simulink model "Non_Holonomical_Cubli"  (R2025b)
settings: Solver=ode15s  StartTime=0  StopTime=13  MaxStep=1e-3  MinStep=1e-8  RelTol=1e-3
values from neighbouring files (symbols this model uses):
  m = 1.219    [physical_parameters.mat]    (also in tuning_parameter_corner.mat; tuning_parameter_edge.mat)
undefined symbols (not defined in the file or in its folder): X, Y, Z
libraries: sm_lib x79, nesl_utility x10, simulink x5, simulink_extras x2
(part 3 of 3)

== system Non_Holonomical_Cubli/Cubli System/Cubli/Non-Motor frame setup/Nonmotor frame 3/Frame ==
  Regular frame : sm_lib/Body Elements/File Solid  ExtGeomFileName=D:\Mechatronics\Non-Holonomical Cubli\GitHub Referance\balancing-cube-main\mechanical\models\frame-regular.step  UnitType=FromFile  ExtGeomFileUnits=m  StepReaderType=HEX  ExportConvexHullGeometry=off  InertiaType=Custom  BasedOnType=DensityFromFile  Density=1000  DensityUnits=kg/m^3  Mass=27.912  MassUnits=g  CenterOfMass=[75.00 75.00 1.481]  CenterOfMassUnits=mm  MomentsOfInertia=[8.5196926e-5 5.2659387e-5 1.378e-4]  MomentsOfInertiaUnits=kg*m^2  ProductsOfInertia=[0 0 0]  ProductsOfInertiaUnits=kg*m^2  GraphicType=FromGeometry  MarkerShape=Sphere  MarkerSize=10  GraphicVisPropType=SimpleVisualProperties  GraphicDiffuseColor=[0 0.5137 0.8314]  GraphicOpacity=1  GraphicSpecularColor=[0.5 0.5 0.5 1.0]  GraphicAmbientColor=[0.15 0.15 0.15 1.0]  GraphicEmissiveColor=[0.0 0.0 0.0 1.0]  GraphicShininess=75  DoExposeReferenceFrame=on  SerializedFrames=<Frames/>
  World to frame : sm_lib/Frames and Transforms/Rigid Transform  RotationMethod=None  FollAlignAxisA=+X  BaseAlignAxisA=+Y  FollAlignAxisB=+Y  BaseAlignAxisB=+Z  RotationStandardAxis=+Z  RotationAngle=0  RotationAngleUnits=deg  RotationArbitraryAxis=[0 0 1]  RotationSequenceAxes=FollowerAxes  RotationSequence=XYX  RotationSequenceAngles=[0 0 0]  RotationSequenceAnglesUnits=deg  RotationMatrix=[1 0 0;0 1 0;0 0 1]  Quaternion=[1 0 0 0]  TranslationMethod=Cartesian  TranslationCartesianOffset=[-75 -75 0]  TranslationCartesianOffsetUnits=mm  TranslationStandardAxis=+Z  TranslationStandardOffset=7  TranslationStandardOffsetUnits=mm  TranslationROffset=0  TranslationROffsetUnits=m  TranslationThetaOffset=0  TranslationThetaOffsetUnits=deg  TranslationZOffset=0  TranslationZOffsetUnits=m
  W to F : PMIOPort  Side=Left
  connections:
  W to F/RConn1 -- World to frame/LConn1
  Regular frame/RConn1 -- World to frame/RConn1

== system Non_Holonomical_Cubli/Cubli System/Cubli/Non-Motor frame setup/Nonmotor frame 3/PCB setup ==
  Frame to PCB : sm_lib/Frames and Transforms/Rigid Transform  RotationMethod=None  FollAlignAxisA=+X  BaseAlignAxisA=+Y  FollAlignAxisB=+Y  BaseAlignAxisB=+Z  RotationStandardAxis=+Z  RotationAngle=0  RotationAngleUnits=deg  RotationArbitraryAxis=[0 0 1]  RotationSequenceAxes=FollowerAxes  RotationSequence=XYX  RotationSequenceAngles=[0 0 0]  RotationSequenceAnglesUnits=deg  RotationMatrix=[1 0 0;0 1 0;0 0 1]  Quaternion=[1 0 0 0]  TranslationMethod=Cartesian  TranslationCartesianOffset=[0 0 -12]  TranslationCartesianOffsetUnits=mm  TranslationStandardAxis=+Z  TranslationStandardOffset=0  TranslationStandardOffsetUnits=m  TranslationROffset=0  TranslationROffsetUnits=m  TranslationThetaOffset=0  TranslationThetaOffsetUnits=deg  TranslationZOffset=0  TranslationZOffsetUnits=m
  PCB : sm_lib/Body Elements/Brick Solid  BrickDimensions=[95 95 15]  BrickDimensionsUnits=mm  ExportEntireGeometry=off  InertiaType=CalculateFromGeometry  BasedOnType=Mass  Density=1000  DensityUnits=kg/m^3  Mass=138.5  MassUnits=g  CenterOfMass=[0 0 0]  CenterOfMassUnits=mm  MomentsOfInertia=[8.25e-5 8.25e-5 1.485e-4]  MomentsOfInertiaUnits=kg*m^2  ProductsOfInertia=[0 0 0]  ProductsOfInertiaUnits=kg*m^2  GraphicType=FromGeometry  MarkerShape=Sphere  MarkerSize=10  GraphicVisPropType=SimpleVisualProperties  GraphicDiffuseColor=[0.5922 0 0.9608]  GraphicOpacity=1  GraphicSpecularColor=[0.5 0.5 0.5 1.0]  GraphicAmbientColor=[0.15 0.15 0.15 1.0]  GraphicEmissiveColor=[0.0 0.0 0.0 1.0]  GraphicShininess=75  DoExposeReferenceFrame=on  SerializedFrames=<Frames/>
  F to P : PMIOPort  Side=Left
  connections:
  PCB/RConn1 -- Frame to PCB/RConn1
  Frame to PCB/LConn1 -- F to P/RConn1

== matlab function Non_Holonomical_Cubli/Master Controller/Corner_Balance_Torque/quaternion_corner_controller ==
  settings: sampleTime=0.00001
  data: q_current input; tau_x output; omega_frame input; omega_wheels input; jump_tigger input; tau_y output; tau_z output; tau_y_edge input; q_ev_corner output; error_distance output
function [tau_x, tau_y, tau_z, q_ev_corner, error_distance] = quaternion_corner_controller(q_current, omega_frame, omega_wheels, jump_tigger, tau_y_edge)
    % q_current:    [w, x, y, z] live orientation from the IMU/Sensor
    % omega_frame:  [wx, wy, wz] in rad/s from the gyroscope (Body Frame)
    % omega_wheels: [wx_wheel, wy_wheel, wz_wheel] in rad/s

    tau_x = 0;
    tau_y = 0;
    tau_z = 0;

    % =========================================================
    % 1. PHYSICAL CONSTANTS
    % =========================================================
    I_matrix = [0.01757, -0.00664, -0.00656; 
               -0.00664,  0.01757, -0.00656; 
               -0.00656, -0.00656,  0.01757];
               
    I_wheel = 0.0005148;     
    m = 1.219;           
    g = 9.80665;            
    r_com = [0.0724; 0.0724; 0.0724]; 

    % =========================================================
    % 2. TARGET ORIENTATIONS (Pre-calculated Quaternions)
    % =========================================================
    % A. The True Corner (Roll = 45 deg, Pitch = -35.26 deg, Yaw = 0)
    % Taken exactly from your previously successful sensor readings
    q_target_corner = [0.8805, 0.2798, -0.3647, -0.1159];
    
    % =========================================================
    % 3. ERROR CALCULATION & UNWINDING FIX (Hamilton Product)
    % =========================================================
    % Extract current quaternion components for readability
    wc = q_current(1); xc = q_current(2); yc = q_current(3); zc = q_current(4);
    
    % --- Calculate Error for the CORNER ---
    % q_error = q_target_corner_inverse * q_current
    w1_c = q_target_corner(1); x1_c = -q_target_corner(2); y1_c = -q_target_corner(3); z1_c = -q_target_corner(4);
    
    q_ew_c = w1_c*wc - x1_c*xc - y1_c*yc - z1_c*zc;
    q_ex_c = w1_c*xc + x1_c*wc + y1_c*zc - z1_c*yc;
    q_ey_c = w1_c*yc - x1_c*zc + y1_c*wc + z1_c*xc;
    q_ez_c = w1_c*zc + x1_c*yc - y1_c*xc + z1_c*wc;
    
    % Shortest path enforcement (Unwinding Fix)
    if q_ew_c < 0
        q_ew_c = -q_ew_c; q_ex_c = -q_ex_c; q_ey_c = -q_ey_c; q_ez_c = -q_ez_c;
    end
    q_ev_corner = [q_ex_c; q_ey_c; q_ez_c];
    
    % Check how close the cube is to the 3D corner (Vector Magnitude)
    error_distance = norm(q_ev_corner);

    % =========================================================
    % 4. STATE MACHINE (Edge to Corner Logic)
    % =========================================================

    if jump_tigger > 0.0 && jump_tigger < 2.0
        % ---------------------------------------------------------
        % STATE 1: THE X-AXIS TORQUE BUILD UP
        % ---------------------------------------------------------
        jump_torque_x =  0.15; % Fire the X-wheel upward
        jump_torque_z = -0.15; % Fire the Z-wheel upward
        
        tau_motor = [jump_torque_x; tau_y_edge; jump_torque_z];

        tau_x = tau_motor(1);
        tau_y = tau_motor(2);
        tau_z = tau_motor(3);

    elseif jump_tigger >= 2.0 && jump_tigger < 2.02
        % ---------------------------------------------------------
        % STATE 2: THE X-AXIS JUMP
        % ---------------------------------------------------------
        jump_torque_x = -14.5; % Fire the X-wheel upward
        jump_torque_z =  14.5; % Fire the Z-wheel upward
        
        tau_motor = [jump_torque_x; 0; jump_torque_z];

        tau_x = tau_motor(1);
        tau_y = tau_motor(2);
        tau_z = tau_motor(3);
        
    elseif jump_tigger >= 2.032 && error_distance <= 0.075

        % ---------------------------------------------------------
        % STATE 3: SMC 3D CORNER CATCH & BALANCE
        % ---------------------------------------------------------
        c = diag([30, 30, 30]);      
        K = [1.5; 1.5; 1.5];             
        epsilon = 0.1; 
        
        % A. Exact Quaternion Derivative for alpha_desired
        q_ev_dot = 0.5 * (q_ew_c * omega_frame + cross(q_ev_corner, omega_frame));
        
        % B. The 3D Sliding Surface
        S = (c * q_ev_corner) + omega_frame;
        
        % C. Dynamic Gravity Compensation (Using Quaternion to DCM rotation)
        % Extracts the 3rd Row of the rotation matrix using live quaternion values
        R31 = 2 * (xc*zc - wc*yc);
        R32 = 2 * (yc*zc + wc*xc);
        R33 = 1 - 2 * (xc^2 + yc^2);
        
        g_body_rotated = [-g * R31; -g * R32; -g * R33];
        tau_gravity = cross(r_com, m * g_body_rotated);
        
        % D. SMC Equivalent Control (tau_eq)
        L_wheels = I_wheel .* omega_wheels; 
        alpha_desired = -c * q_ev_dot;
        
        tau_eq = - (I_matrix * alpha_desired) - cross(omega_frame, (I_matrix * omega_frame + L_wheels)) - tau_gravity;
                 
        % E. SMC Switching Control (tau_sw)
        tau_sw = -K .* tanh(S / epsilon);
        
        % F. Total Torque (Newton's Third Law flipped)
        tau_frame = tau_eq + tau_sw;
        tau_motor = -tau_frame;

        % G. Motor Saturation
        max_torque = 1.2;
        tau_x = max(min(tau_motor(1), max_torque), -max_torque);
        tau_y = max(min(tau_motor(2), max_torque), -max_torque);
        tau_z = max(min(tau_motor(3), max_torque), -max_torque);
    end 
end

== matlab function Non_Holonomical_Cubli/Master Controller/Edge_Balance_Torque/Edge_SMC ==
  data: tau_x output; theta_current input; omega_frame input; omega_wheels input; tau_y output; tau_z output; error_distance output; jump_trigger input
function [tau_x, tau_y, tau_z,error_distance] = smc_edge_controller(theta_current, omega_frame, omega_wheels, jump_trigger)
    % theta_current: [roll, pitch, yaw] in radians from the sensor (Earth Frame)
    % omega_frame:   [wx, wy, wz] in rad/s from the gyroscope (Body Frame)
    % omega_wheels:  [wx_wheel, wy_wheel, wz_wheel] in rad/s

    jump_check = 0;
    tau_motor = [0; 0; 0;];

    % =========================================================
    % 1. PHYSICAL CONSTANTS (Matches your CAD parameters)
    % =========================================================
    I_matrix = [0.01757, -0.00664, -0.00656; 
               -0.00664,  0.01757, -0.00656; 
               -0.00656, -0.00656,  0.01757];
               
    I_wheel = 0.0005148;     % Inertia of a single brass wheel (kg*m^2)
    m = 1.291;           % Total mass (kg)
    g = 9.80665;            % Gravity (m/s^2)
    
    % True Center of Mass vector from the EDGE pivot
    r_com = [0.0724; 0.0724; 0.0724]; 

    % =========================================================
    % 2. OUTER LOOP: MOMENTUM MANAGEMENT (Deadband Lean)
    % =========================================================
    % We apply a proportional shift ONLY if the wheel exceeds the safe zone.
    safe_speed = 200;  % ~1000 RPM in rad/s
    k_momentum = 1e-4; % Gain: How much to lean per rad/s over the limit
    max_lean = 0.0167*3;     % Safety limit: Max lean of ~1 degrees

    % Read instantaneous Y-axis (Pitch) wheel speed
    pitch_wheel_speed = omega_wheels(2);

    % Deadband logic
    if pitch_wheel_speed > safe_speed
        active_omega = pitch_wheel_speed - safe_speed;
    elseif pitch_wheel_speed < -safe_speed
        active_omega = pitch_wheel_speed + safe_speed;
    else
        active_omega = 0; % Inside safe zone, do not lean
    end 

    % Calculate and saturate the lean shift
    lean_shift = k_momentum * active_omega;
    lean_shift = max(min(lean_shift, max_lean), -max_lean);

    % Generate dynamic target (Base -45 deg edge + shift)
    target_pitch = -0.7854 - lean_shift;
    theta_target = [0; target_pitch; 0];
    
    % =========================================================
    % 3. CALCULATE ERRORS & FRAME MAPPING
    % =========================================================
    % Raw Position error (In Earth Frame)
    e_euler = theta_current - theta_target;
    
    % Extract current Roll (phi) and Pitch (theta)
    phi = theta_current(1);
    theta = theta_current(2);
    
    % Kinematic Transformation Matrix (W)
    % Maps Earth-frame Euler angle errors into physical Body-frame axes
    W = [1,  0,        -sin(theta); 
         0,  cos(phi),  sin(phi)*cos(theta); 
         0, -sin(phi),  cos(phi)*cos(theta)];
         
    % Project the error into the physical Body Frame
    e_body = W * e_euler;
    e_dot_body = omega_frame;
    
    % Check how close the cube is to the edge balance point (in radians)
    error_distance = norm(e_body);

    % =========================================================
    % 4. SMC 3D EDGE CATCH & BALANCE
    % =========================================================
    if jump_trigger >= 0.2 && jump_trigger <= 2.3
        % ---------------------------------------------------------
        % STATE 1: THE Y-AXIS TORQUE BUILD UP
        % ---------------------------------------------------------
        tau_motor = [0; -0.2; 0];

        jump_check = 0;

    elseif jump_trigger >= 2.3 && jump_trigger <= 2.32
        % ---------------------------------------------------------
        % STATE 2: THE Y-AXIS JUMP
        % ---------------------------------------------------------
        tau_motor = [0; 21; 0];

        jump_check = 1;

    elseif jump_trigger >= 2.32 && theta <= -0.3927
        % A. SMC Tuning Parameters
        c = 30;        % Sliding surface slope (Urgency)
        K = 0.8;       % Switching gain (Muscle)
        epsilon = 0.1; % Boundary layer (Smooths out chattering)
        
        % B. The 3D Sliding Surface (3x1 Vector)
        S = (c * e_body) + e_dot_body;
        
        % C. Dynamic Gravity Compensation (Rotate World Z down to Body)
        R31 = -sin(theta);
        R32 = cos(theta) * sin(phi);
        R33 = cos(theta) * cos(phi);
        g_body_rotated = [-g * R31; -g * R32; -g * R33];
        tau_gravity = cross(r_com, m * g_body_rotated);
        
        % D. SMC Equivalent Control (tau_eq)
        L_wheels = I_wheel .* omega_wheels; 
        alpha_desired = -c * e_dot_body;
        
        % Full 3D Inverse Dynamics
        tau_eq = (I_matrix * alpha_desired) + cross(omega_frame, (I_matrix * omega_frame + L_wheels)) - tau_gravity;
                 
        % E. SMC Switching Control (tau_sw)
        tau_sw = -K * tanh(S / epsilon);
        
        % F. Total Torque (Newton's Third Law flipped for the motors)
        tau_frame = tau_eq + tau_sw;
        tau_motor = [0; -tau_frame(2); 0];
        
        jump_check = 0;
        
    end

    % =========================================================
    % 5. OUTPUT ASSIGNMENT & SATURATION
    % =========================================================
    
    tau_x = tau_motor(1);
    tau_z = tau_motor(3);

    if jump_check == 1

        tau_y = tau_motor(2);

    else

        % Limit the motors to their physical maximum (e.g. 1.2 N-m)
        max_torque = 1.2;
        tau_y = max(min(tau_motor(2), max_torque), -max_torque);

    end
